simulink model "Lab4_Lag"  (R2016a)
settings: Solver=VariableStepAuto  StartTime=0.0  StopTime=20  RelTol=1e-3
settings Model: Creator=jordan  LastModifiedBy=jordan

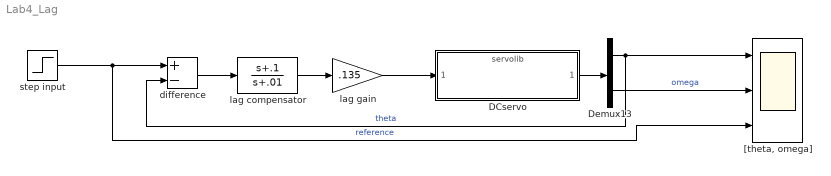
== system Lab4_Lag ==
  DCservo : ModelReference  ModelNameDialog=servolib.slx  SimulationMode=Normal  ModelReferenceVersion=1.77
  Demux13 : Demux  Outputs=2
  "[theta, omega]" : Scope  NumInputPorts=3
  difference : Sum  Inputs=+-
  lag compensator : TransferFcn  Numerator=[1 .1]  Denominator=[1 .01]
  lag gain : Gain  Gain=.135
  step input : Step  SampleTime=0
  wires:
  Demux13/2 -> "[theta, omega]"/2  "omega"
  difference/1 -> lag compensator/1
  Demux13/1 -> "[theta, omega]"/1, difference/2  "theta"
  step input/1 -> "[theta, omega]"/3, difference/1  "reference"
  lag compensator/1 -> lag gain/1
  lag gain/1 -> DCservo/1
  DCservo/1 -> Demux13/1
